simulink model "projekt1"  (R2018b)
settings: Solver=VariableStepAuto  StartTime=0.0  StopTime=100  RelTol=1e-3
undefined symbols (not defined in the file or in its folder): sigbuilder_block
libraries: simulink_extras x1, commrandsrc3 x1
settings Model: Creator=michask  LastModifiedBy=michask

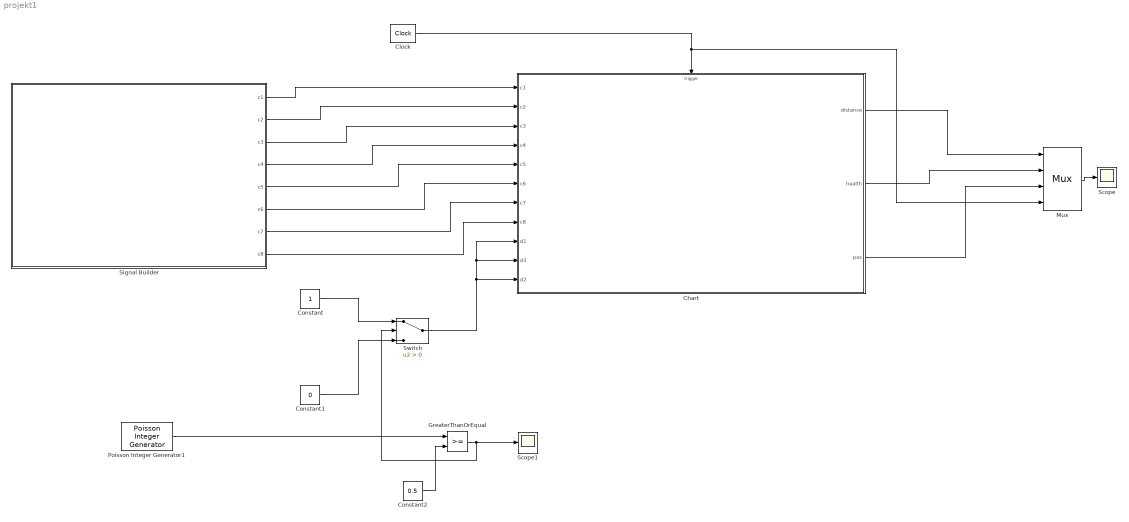
== system projekt1 ==
  Chart : Stateflow chart  TreatAsAtomicUnit=on
  Clock : simulink_extras/Flip Flops/Clock  period=0.1
  Constant : Constant
  Constant1 : Constant  Value=0
  Constant2 : Constant  Value=0.5
  GreaterThanOrEqual : RelationalOperator  OutDataTypeStr=boolean  RndMeth=Simplest
  Mux : Mux
  Poisson Integer Generator1 : commrandsrc3/Poisson Integer Generator  PoissonParameter=0.05  SeedSource=Auto  Seed=0  SampleTime=0.1  SamplesPerFrame=1  OutputDataType=double  SimulateUsing=Interpreted execution
      settings: SourceProductName=Communications System Toolbox  SourceProductBaseCode=CM
  Scope : Scope
  Scope1 : Scope
  Signal Builder : Subsystem  Tag=STV Subsys  LoadFcn=sigbuilder_block('load');  StartFcn=sigbuilder_block('start');  StopFcn=sigbuilder_block('stop');  ClipboardFcn=sigbuilder_block('clipboard');  mask(Sigbuilder block){tuvar=[0:10]}
      mask help: Simulink:masks:SigbuilderBlock_MD
      mask init:
      | if ~strcmp(get_param(bdroot(gcbh),'SimulationStatus'),'stopped') tuvar = sigbuilder_block('maskInit'); end
      settings: CopyFcn=sigbuilder_block('copy');  DeleteFcn=sigbuilder_block('delete');  ModelCloseFcn=sigbuilder_block('modelClose');  PreSaveFcn=sigbuilder_block('preSave');  PauseFcn=sigbuilder_block('pause');  ContinueFcn=sigbuilder_block('continue');  NameChangeFcn=sigbuilder_block('namechange');  OpenFcn=sigbuilder_block('open',[437.6 199.2 550.4 400 ]);  CloseFcn=sigbuilder_block('close');
      mask Display: plot(0, 0, 100, 100,[2, 2, 32, 32, 2], [68, 8, 8, 68, 68],[32, 2], [38, 38], [32, 19, 2],[53, 60, 44], [32, 17, 17, 2],[16, 16, 31, 31]);txt = getActiveGroup(gcbh);text(2, 100, txt,'verticalAlignment', 'top');
  Switch : Switch  Criteria=u2 > Threshold
  wires:
  Signal Builder/5(c5) -> Chart/5(c5)
  Signal Builder/1(c1) -> Chart/1(c1)
  Signal Builder/2(c2) -> Chart/2(c2)
  Signal Builder/3(c3) -> Chart/3(c3)
  Signal Builder/4(c4) -> Chart/4(c4)
  Signal Builder/6(c6) -> Chart/6(c6)
  Signal Builder/7(c7) -> Chart/7(c7)
  Signal Builder/8(c8) -> Chart/8(c8)
  Chart/1(distance) -> Mux/1
  Chart/2(health) -> Mux/2
  Chart/3(pos) -> Mux/3
  Mux/1 -> Scope/1
  Clock/1 -> Chart/Trigger, Mux/4
  Switch/1 -> Chart/11(d2), Chart/10(d3), Chart/9(d1)
  Constant1/1 -> Switch/3
  Constant/1 -> Switch/1
  Constant2/1 -> GreaterThanOrEqual/2
  Poisson Integer Generator1/1 -> GreaterThanOrEqual/1
  GreaterThanOrEqual/1 -> Scope1/1, Switch/2

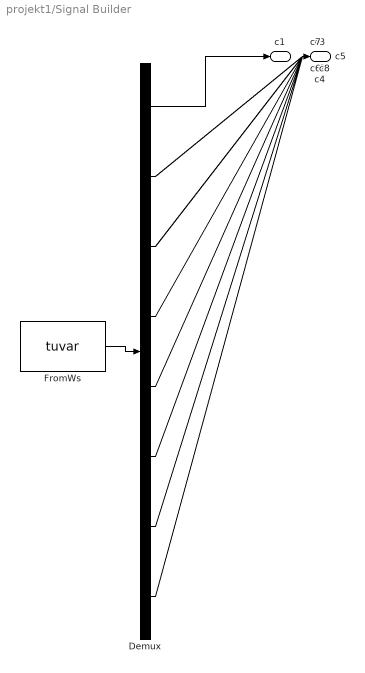
== system projekt1/Signal Builder ==
  Demux : Demux  Tag=STV Demux  Outputs=8
  FromWs : FromWorkspace  Tag=STV FromWs  VariableName=tuvar  SampleTime=0
      SigBuilderData=|
      | common.afterFinalStr = 'Extrapolate'
      | common.sampleTime = 0
      | dataSet.timeRange = [0 10]
      | dataSet.name = 'Group 1'
      | sbobj.Groups.Name = 'Group 1'
      | sbobj.Groups.Signals(1).Name = 'c1'
      | sbobj.Groups.Signals(1).XData = [0 4 4 6 6 10]
      | sbobj.Groups.Signals(1).YData = [0 -0.1 1 1 0 0]
      | sbobj.Groups.Signals(2).Name = 'c2'
      | sbobj.Groups.Signals(2).XData = [0 4 4 6 6 10]
      | sbobj.Groups.Signals(2).YData = [0 0 1 1 0 0]
      | sbobj.Groups.Signals(3).Name = 'c3'
      | sbobj.Groups.Signals(3).XData = [0 4 4 6 6 10]
      | sbobj.Groups.Signals(3).YData = [0 0 1 1 0 0]
      | sbobj.Groups.Signals(4).Name = 'c4'
      | sbobj.Groups.Signals(4).XData = [0 4 4 6 6 10]
      | sbobj.Groups.Signals(4).YData = [0 0 1 1 0 0]
      | sbobj.Groups.Signals(5).Name = 'c5'
      | sbobj.Groups.Signals(5).XData = [0 4 4 6 6 10]
      | sbobj.Groups.Signals(5).YData = [0 0 1 1 0 0]
      | sbobj.Groups.Signals(6).Name = 'c6'
      | sbobj.Groups.Signals(6).XData = [0 4 4 6 6 10]
      | sbobj.Groups.Signals(6).YData = [0 0 1 1 0 0]
      | sbobj.Groups.Signals(7).Name = 'c7'
      | sbobj.Groups.Signals(7).XData = [0 4 4 6 6 10]
      | sbobj.Groups.Signals(7).YData = [0 0 1 1 0 0]
      | sbobj.Groups.Signals(8).Name = 'c8'
      | sbobj.Groups.Signals(8).XData = [0 4 4 6 6 10]
      | sbobj.Groups.Signals(8).YData = [0 0 1 1 0 0]
  c1 : Outport  Tag=STV Outport
  c2 : Outport  Tag=STV Outport  Port=2
  c3 : Outport  Tag=STV Outport  Port=3
  c4 : Outport  Tag=STV Outport  Port=4
  c5 : Outport  Tag=STV Outport  Port=5
  c6 : Outport  Tag=STV Outport  Port=6
  c7 : Outport  Tag=STV Outport  Port=7
  c8 : Outport  Tag=STV Outport  Port=8
  wires:
  Demux/1 -> c1/1
  FromWs/1 -> Demux/1
  Demux/2 -> c2/1
  Demux/3 -> c3/1
  Demux/4 -> c4/1
  Demux/5 -> c5/1
  Demux/6 -> c6/1
  Demux/7 -> c7/1
  Demux/8 -> c8/1

== stateflow chart projekt1/Chart ==
  settings: executeAtInitialization=1
  state M
  state H
    en:
    t=t+1
    p3=rand
  state P
    en:
    t=t+1
  state E%eksploracja
    en:
    p1=rand
    p2=rand
    p4=rand
    kierunek = rand
    t=t+1
    if distance < 2*pi
    if kierunek > 0.15
    distance = distance + 3.14/4
    else distance = distance - 3.14/4
    end
    else
    distance = 3.14/4
    end
  state D
  state C
    en:
    p9=rand
  state F
  state W
  state R
    en:
    p5=rand
    p7=rand
    t=t+1
  P -> H : [c1]
  H -> D : [p3>r3]
  E%eksploracja -> P [order 3] : [p1<r1]
  (default) -> E%eksploracja
  E%eksploracja -> D [order 1] : [p2<r2]
  D -> C : [d1]
  C -> R : [p9>r9]
  E%eksploracja -> R [order 4] : [p4>r4]
  E%eksploracja -> E%eksploracja [order 2] : [clock]
  data: c1 input; c2 input; c3 input; c4 input; c5 input; c6 input; c7 input; c8 input; distance output =0; health output =1; pos output =0; d1 input; d3 input; d2 input; p2 local; r2 local =0.8; t local =0; r3 local =0.2; p3 local; r10 local; r9 local =0.01; r8 local; r7 local; r6 local =0.01; r5 local; r4 local =0.01; r11 local; r12 local; p4 local; p5 local; p6 local; p7 local; p8 local; p9 local; p10 local; p11 local; p12 local; kierunek local; r1 local =1/8; p1 local
  events: clock input RISING_EDGE_EVENT
